simulink model "PID_Controller"  (R2017b)
settings: Solver=VariableStepAuto  StartTime=0.0  StopTime=10.0  RelTol=1e-3  EnableMultiTasking=on
undefined symbols (not defined in the file or in its folder): Fmatrix, Imatrix
libraries: dspinverses x1
(part 1 of 5)
settings Model: Creator=as01398  LastModifiedBy=jedmcinnes
settings DataIOCC: OutputOption=SpecifiedOutputTimes  OutputTimes=[0:0.2:10]
settings OptimizationCC: LifeSpan=inf
settings DebuggingCC: SFUnexpectedBacktrackingDiag=warning  SFNoUnconditionalDefaultTransitionDiag=warning  SFExecutionAtInitializationDiag=none
settings CodeAppCC: StateflowObjectComments=on
settings GRTTargetCC: TargetLangStandard=C89/C90 (ANSI)  GeneratePreprocessorConditionals=Disable all
settings ConfigComp: CovMetricSettings=dw  CovHtmlReporting=on  CovSaveCumulativeToWorkspaceVar=on  CovSaveSingleToWorkspaceVar=on  CovExternalEMLEnable=off

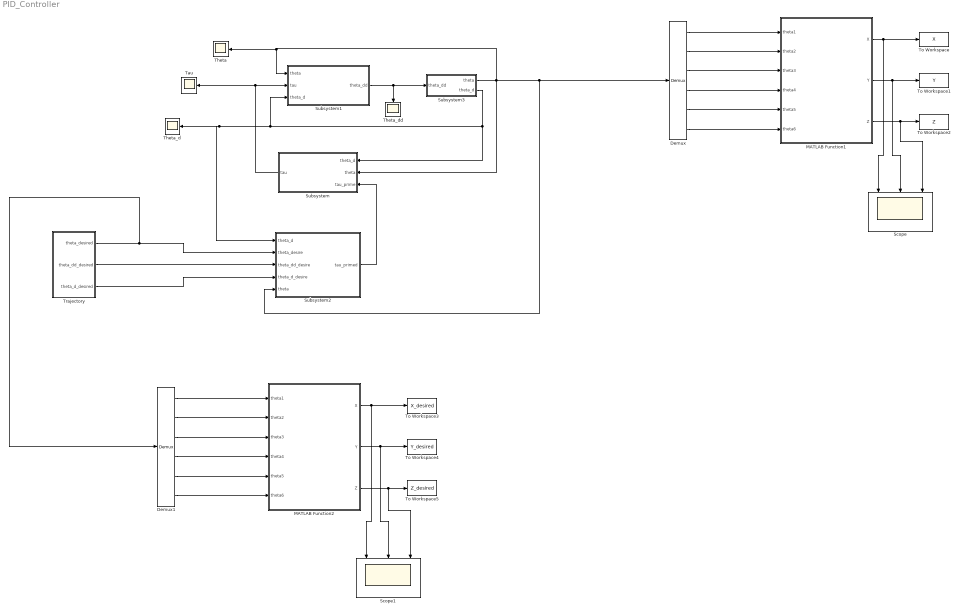
== system PID_Controller ==
  Demux : Demux  Outputs=6
  Demux1 : Demux  Outputs=6
  MATLAB Function1 : MATLAB Function  TreatAsAtomicUnit=on
  MATLAB Function2 : MATLAB Function  TreatAsAtomicUnit=on
  Scope : Scope  NumInputPorts=3
  Scope1 : Scope  NumInputPorts=3
  Subsystem : Subsystem
  Subsystem1 : Subsystem
  Subsystem2 : Subsystem
  Subsystem3 : Subsystem
  Tau : Scope
  Theta : Scope
  Theta_d : Scope
  Theta_dd : Scope
  To Workspace : ToWorkspace  VariableName=X  SampleTime=-1
  To Workspace1 : ToWorkspace  VariableName=Y  SampleTime=-1
  To Workspace2 : ToWorkspace  VariableName=Z  SampleTime=-1
  To Workspace3 : ToWorkspace  VariableName=X_desired  SampleTime=-1
  To Workspace4 : ToWorkspace  VariableName=Y_desired  SampleTime=-1
  To Workspace5 : ToWorkspace  VariableName=Z_desired  SampleTime=-1
  Trajectory : Subsystem
  wires:
  Demux/2 -> MATLAB Function1/2(theta2)
  Demux/1 -> MATLAB Function1/1(theta1)
  Demux/3 -> MATLAB Function1/3(theta3)
  Demux/4 -> MATLAB Function1/4(theta4)
  Demux/5 -> MATLAB Function1/5(theta5)
  Demux/6 -> MATLAB Function1/6(theta6)
  MATLAB Function1/3(Z) -> Scope/3, To Workspace2/1
  MATLAB Function1/2(Y) -> Scope/2, To Workspace1/1
  Subsystem/1(tau) -> Subsystem1/2(tau), Tau/1
  Subsystem2/1(tau_primed) -> Subsystem/3(tau_prime)
  Trajectory/2(theta_dd_desired) -> Subsystem2/3(theta_dd_desire)
  Trajectory/3(theta_d_desired) -> Subsystem2/4(theta_d_desire)
  Subsystem1/1(theta_dd) -> Theta_dd/1, Subsystem3/1(theta_dd)
  Subsystem3/2(theta_d) -> Subsystem1/3(theta_d), Theta_d/1, Subsystem2/1(theta_d), Subsystem/1(theta_d)
  MATLAB Function1/1(X) -> Scope/1, To Workspace/1
  Subsystem3/1(theta) -> Demux/1, Subsystem2/5(theta), Subsystem/2(theta), Theta/1, Subsystem1/1(theta)
  Demux1/2 -> MATLAB Function2/2(theta2)
  MATLAB Function2/2(Y) -> Scope1/2, To Workspace4/1
  MATLAB Function2/1(X) -> Scope1/1, To Workspace3/1
  Demux1/1 -> MATLAB Function2/1(theta1)
  Demux1/3 -> MATLAB Function2/3(theta3)
  Demux1/5 -> MATLAB Function2/5(theta5)
  Demux1/6 -> MATLAB Function2/6(theta6)
  Demux1/4 -> MATLAB Function2/4(theta4)
  MATLAB Function2/3(Z) -> Scope1/3, To Workspace5/1
  Trajectory/1(theta_desired) -> Demux1/1, Subsystem2/2(theta_desire)

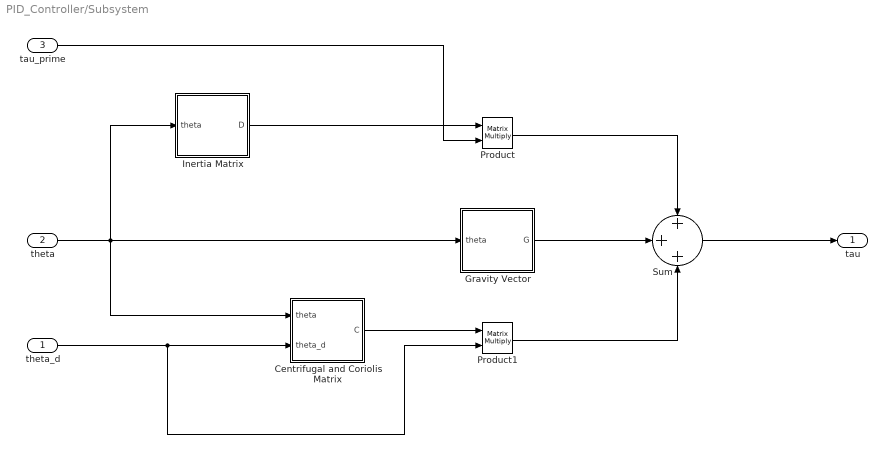
== system PID_Controller/Subsystem ==
  theta_d : Inport
  theta : Inport  Port=2
  tau_prime : Inport  Port=3
  Centrifugal and Coriolis Matrix : Subsystem
  Gravity Vector : Subsystem
  Inertia Matrix : Subsystem
  Product : Product  Multiplication=Matrix(*)
  Product1 : Product  Multiplication=Matrix(*)
  Sum : Sum  Inputs=+++
  tau : Outport
  wires:
  theta/1 -> Gravity Vector/1(theta), Inertia Matrix/1(theta), Centrifugal and Coriolis Matrix/1(theta)
  Inertia Matrix/1(D) -> Product/1
  tau_prime/1 -> Product/2
  theta_d/1 -> Product1/2, Centrifugal and Coriolis Matrix/2(theta_d)
  Centrifugal and Coriolis Matrix/1(C) -> Product1/1
  Product/1 -> Sum/1
  Gravity Vector/1(G) -> Sum/2
  Product1/1 -> Sum/3
  Sum/1 -> tau/1

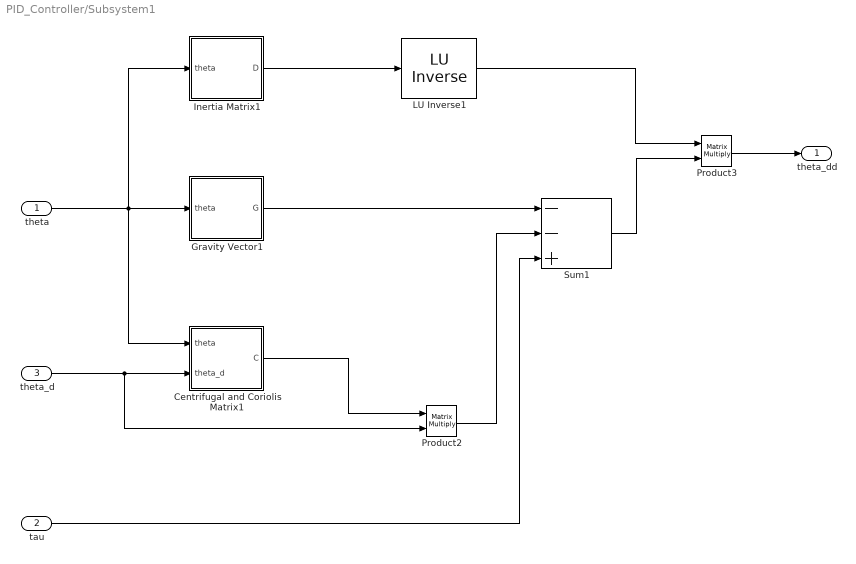
== system PID_Controller/Subsystem1 ==
  theta : Inport
  tau : Inport  Port=2
  theta_d : Inport  Port=3
  " LU Inverse1" : dspinverses/ LU Inverse
      settings: SourceProductName=DSP System Toolbox
  Centrifugal and Coriolis Matrix1 : Subsystem
  Gravity Vector1 : Subsystem
  Inertia Matrix1 : Subsystem
  Product2 : Product  Multiplication=Matrix(*)
  Product3 : Product  Multiplication=Matrix(*)
  Sum1 : Sum  Inputs=--+
  theta_dd : Outport
  wires:
  theta/1 -> Centrifugal and Coriolis Matrix1/1(theta), Inertia Matrix1/1(theta), Gravity Vector1/1(theta)
  theta_d/1 -> Product2/2, Centrifugal and Coriolis Matrix1/2(theta_d)
  Centrifugal and Coriolis Matrix1/1(C) -> Product2/1
  Inertia Matrix1/1(D) -> " LU Inverse1"/1
  Product2/1 -> Sum1/2
  Gravity Vector1/1(G) -> Sum1/1
  tau/1 -> Sum1/3
  " LU Inverse1"/1 -> Product3/1
  Sum1/1 -> Product3/2
  Product3/1 -> theta_dd/1

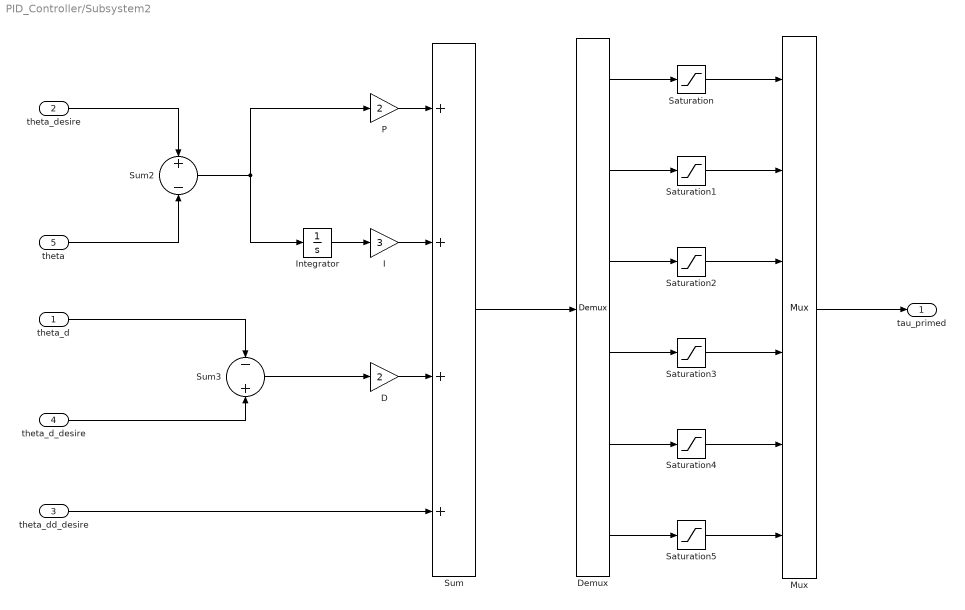
== system PID_Controller/Subsystem2 ==
  theta_d : Inport
  theta_desire : Inport  Port=2
  theta_dd_desire : Inport  Port=3
  theta_d_desire : Inport  Port=4
  theta : Inport  Port=5
  D : Gain  Gain=2
  Demux : Demux  Outputs=6
  I : Gain  Gain=3
  Integrator : Integrator
  Mux : Mux  Inputs=6
  P : Gain  Gain=2
  Saturation : Saturate  UpperLimit=16  LowerLimit=-16
  Saturation1 : Saturate  UpperLimit=32  LowerLimit=-32
  Saturation2 : Saturate  UpperLimit=21  LowerLimit=-21
  Saturation3 : Saturate  UpperLimit=5  LowerLimit=-5
  Saturation4 : Saturate  UpperLimit=5  LowerLimit=-5
  Saturation5 : Saturate  UpperLimit=4  LowerLimit=-4
  Sum : Sum  Inputs=++++
  Sum2 : Sum  Inputs=+-
  Sum3 : Sum  Inputs=-+
  tau_primed : Outport
  wires:
  Sum2/1 -> P/1, Integrator/1
  theta/1 -> Sum2/2
  theta_desire/1 -> Sum2/1
  Integrator/1 -> I/1
  theta_d/1 -> Sum3/1
  theta_d_desire/1 -> Sum3/2
  Sum3/1 -> D/1
  Sum/1 -> Demux/1
  Demux/1 -> Saturation/1
  Demux/2 -> Saturation1/1
  Demux/3 -> Saturation2/1
  Demux/4 -> Saturation3/1
  Demux/5 -> Saturation4/1
  Demux/6 -> Saturation5/1
  Saturation/1 -> Mux/1
  Saturation1/1 -> Mux/2
  Saturation2/1 -> Mux/3
  Saturation3/1 -> Mux/4
  Saturation4/1 -> Mux/5
  Saturation5/1 -> Mux/6
  Mux/1 -> tau_primed/1
  theta_dd_desire/1 -> Sum/4
  D/1 -> Sum/3
  I/1 -> Sum/2
  P/1 -> Sum/1

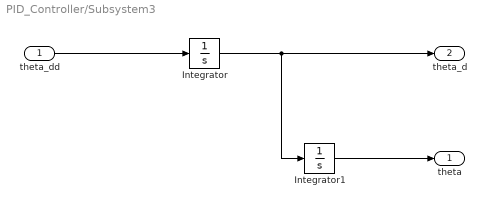
== system PID_Controller/Subsystem3 ==
  theta_dd : Inport
  Integrator : Integrator
  Integrator1 : Integrator
  theta : Outport
  theta_d : Outport  Port=2
  wires:
  theta_dd/1 -> Integrator/1
  Integrator/1 -> Integrator1/1, theta_d/1
  Integrator1/1 -> theta/1

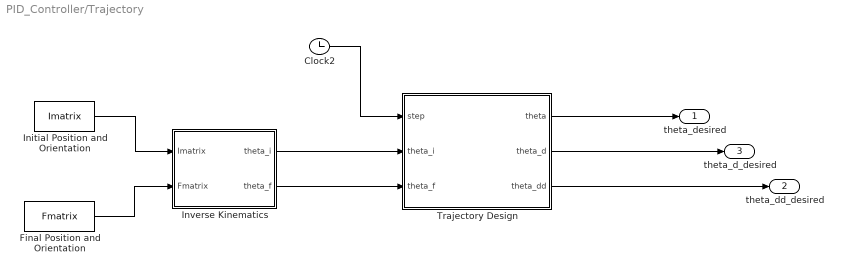
== system PID_Controller/Trajectory ==
  Clock2 : Clock
      settings: Decimation=1000
  Final Position and Orientation : Constant  Value=Fmatrix
  Initial Position and Orientation : Constant  Value=Imatrix
  Inverse Kinematics : MATLAB Function  TreatAsAtomicUnit=on
  Trajectory Design : MATLAB Function  TreatAsAtomicUnit=on
  theta_desired : Outport
  theta_dd_desired : Outport  Port=2
  theta_d_desired : Outport  Port=3
  wires:
  Trajectory Design/3(theta_dd) -> theta_dd_desired/1
  Trajectory Design/2(theta_d) -> theta_d_desired/1
  Trajectory Design/1(theta) -> theta_desired/1
  Inverse Kinematics/2(theta_f) -> Trajectory Design/3(theta_f)
  Inverse Kinematics/1(theta_i) -> Trajectory Design/2(theta_i)
  Final Position and Orientation/1 -> Inverse Kinematics/2(Fmatrix)
  Initial Position and Orientation/1 -> Inverse Kinematics/1(Imatrix)
  Clock2/1 -> Trajectory Design/1(step)

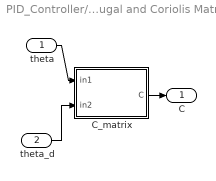
== system PID_Controller/Subsystem/Centrifugal and Coriolis Matrix ==
  theta : Inport
  theta_d : Inport  Port=2
  C_matrix : MATLAB Function  TreatAsAtomicUnit=on
  C : Outport
  wires:
  theta_d/1 -> C_matrix/2(in2)
  theta/1 -> C_matrix/1(in1)
  C_matrix/1(C) -> C/1

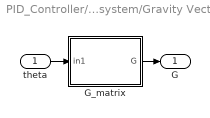
== system PID_Controller/Subsystem/Gravity Vector ==
  theta : Inport
  G_matrix : MATLAB Function  TreatAsAtomicUnit=on
  G : Outport
  wires:
  G_matrix/1(G) -> G/1
  theta/1 -> G_matrix/1(in1)

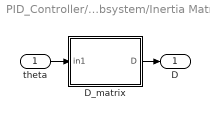
== system PID_Controller/Subsystem/Inertia Matrix ==
  theta : Inport
  D_matrix : MATLAB Function  TreatAsAtomicUnit=on
  D : Outport
  wires:
  D_matrix/1(D) -> D/1
  theta/1 -> D_matrix/1(in1)

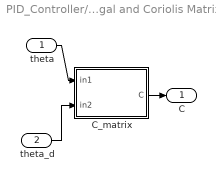
== system PID_Controller/Subsystem1/Centrifugal and Coriolis Matrix1 ==
  theta : Inport
  theta_d : Inport  Port=2
  C_matrix : MATLAB Function  TreatAsAtomicUnit=on
  C : Outport
  wires:
  theta_d/1 -> C_matrix/2(in2)
  theta/1 -> C_matrix/1(in1)
  C_matrix/1(C) -> C/1

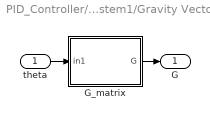
== system PID_Controller/Subsystem1/Gravity Vector1 ==
  theta : Inport
  G_matrix : MATLAB Function  TreatAsAtomicUnit=on
  G : Outport
  wires:
  G_matrix/1(G) -> G/1
  theta/1 -> G_matrix/1(in1)

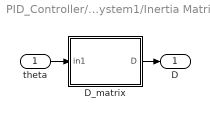
== system PID_Controller/Subsystem1/Inertia Matrix1 ==
  theta : Inport
  D_matrix : MATLAB Function  TreatAsAtomicUnit=on
  D : Outport
  wires:
  D_matrix/1(D) -> D/1
  theta/1 -> D_matrix/1(in1)

== matlab function PID_Controller/MATLAB Function2 ==
  data: theta1 input; X output; theta2 input; theta3 input; theta4 input; theta5 input; theta6 input; Y output; Z output
function [X,Y,Z] = ...
    ForwardKinematic(theta1, theta2, theta3, theta4, theta5, theta6)

    %joint_angles = [theta1,theta2,theta3,theta4,theta5,theta6];
    twist_angles = [-pi/2, 0, pi/2, -pi/2, pi/2, 0];     
    %Note, twist angles should be inputted in radians. 
    link_lengths = [0, 0.5, 0, 0, 0, 0];
    offsets = [0, 0.25, 0, 1, 0, 0.5];
    
    
    A1 = generateAMatrix(theta1,twist_angles(1),link_lengths(1),...
        offsets(1));
    A2 = generateAMatrix(theta2,twist_angles(2),link_lengths(2),...
        offsets(2));
    A3 = generateAMatrix(theta3,twist_angles(3),link_lengths(3),...
        offsets(3));
    A4 = generateAMatrix(theta4,twist_angles(4),link_lengths(4),...
        offsets(4));
    A5 = generateAMatrix(theta5,twist_angles(5),link_lengths(5),...
        offsets(5));
    A6 = generateAMatrix(theta6,twist_angles(6),link_lengths(6),...
        offsets(6));
    
        
    D_H = generateD_HMatrix(A1,A2,A3,A4,A5,A6);
    
    
    X = D_H(1,4);
    Y = D_H(2,4);
    Z = D_H(3,4);
        
end
